simulink model "DGM_test_sim"  (R2020a)
settings: Solver=VariableStepAuto  StartTime=0.0  StopTime=smax  MaxStep=0.01  RelTol=1e-3
values from neighbouring files (symbols this model uses):
  a1 = 2    [OvereniDGMIGM.m]    (also in setup.m)
  a2 = 1.5    [OvereniDGMIGM.m]    (also in setup.m)
  a3 = 0.5    [OvereniDGMIGM.m]    (also in setup.m)
  T_1_0 = [cos(theta10), -sin(theta10), 0, a1*cos(theta10) ... (first row only)    [OvereniDGMIGM.m]    (also in setup.m)
  T_2_1 = [cos(theta20), -sin(theta20), 0, a2*cos(theta20) ... (first row only)    [OvereniDGMIGM.m]    (also in setup.m)
  T_3_2 = [cos(theta30), -sin(theta30), 0, a3*cos(theta30) ... (first row only)    [OvereniDGMIGM.m]    (also in setup.m)
undefined symbols (not defined in the file or in its folder): fi_s, fi_sample, r, R, smax, X, Y, Z
libraries: sm_lib x114, nesl_utility x58, simulink x4
(part 1 of 4)
settings Model: Creator=vilda  LastModifiedBy=Ja
settings DebuggingCC: SFMachineParentedDataDiag=error

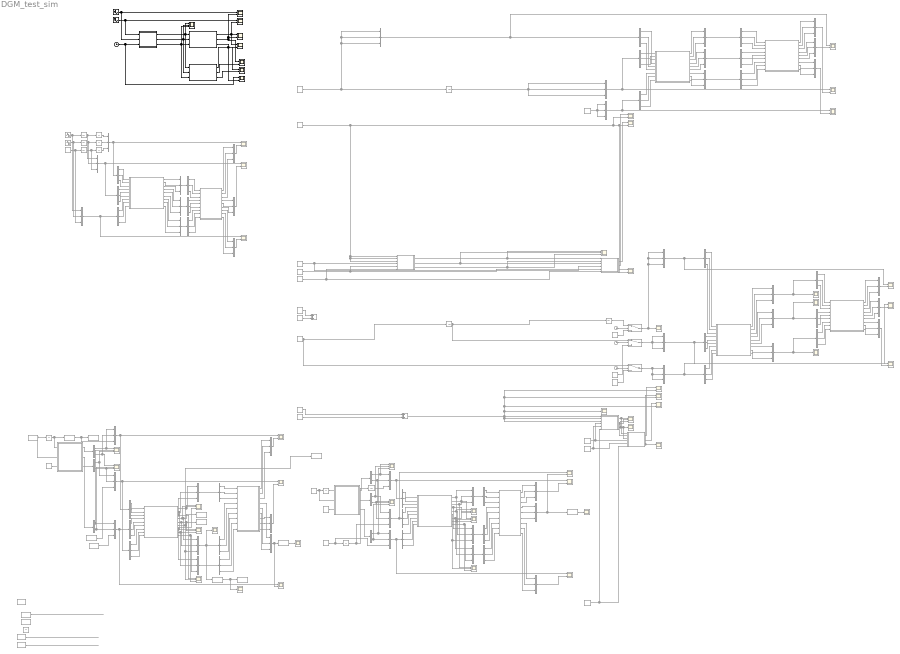
== system DGM_test_sim ==
  note: Kruhova trajektorie
  note: Rychost musi byt mensi nez vmax = 1
  note: IOKU dava manipulatoru polohu, rychlost a zrychleni v kloubech pro docileni polohy, rychlosti a zrychleni v cartezovi
  note: kloubove souradnice
  note: Generator trajektorie
  note: Generator trajektorie
  note: Rychost musi byt mensi nez vmax = 1
  note: Rychost musi byt mensi nez vmax = 1
  Add : Sum  Commented=on
  Add1 : Sum  Commented=on
  Clock : Clock  Commented=on
  Clock1 : Clock  Commented=on
  Clock2 : Clock  Commented=on
  Clock6 : Clock
  Constant{,14,16..17,21..22,24,27..28,30..31} (11 alike) : Constant  Commented=on  Value=0
  Constant10 : Constant  Commented=on  Value=0.6
  Constant11 : Constant  Commented=on  Value=fi_sample
  Constant12 : Constant  Commented=on  Value=0.1  SampleTime=-1
  Constant13 : Constant  Commented=on  Value=0.01  SampleTime=-1
  Constant15 : Constant  Commented=on
  Constant2 : Constant  Commented=on  Value=0  SampleTime=-1
  Constant23 : Constant  Commented=on
  Constant25 : Constant  Commented=on  Value=-fi_s/smax
  Constant29 : Constant  Commented=on  Value=fi_sample
  Constant3 : Constant  Commented=on  Value=a1
  Constant4 : Constant  Commented=on  Value=a2
  Constant5 : Constant  Commented=on  Value=a3
  Constant6 : Constant  Commented=on  Value=a1
  Constant7 : Constant  Commented=on  Value=a2
  Constant8 : Constant  Commented=on  Value=a3
  Demux{,1..23,27..32} (30 alike) : Demux  Commented=on  Outputs=3
  Demux{24..26,33..35} (6 alike) : Demux  Commented=on  Outputs=2
  Fcn : Fcn  Commented=on  Expr=sqrt(u(1)^2+u(2)^2+u(3)^2)
  Fcn1 : Fcn  Commented=on  Expr=sqrt(u(1)^2+u(2)^2+u(3)^2)
  Fcn2 : Fcn  Commented=on  Expr=sqrt(u(1)^2+u(2)^2+u(3)^2)
  Fcn3 : Fcn  Commented=on  Expr=fi_s - fi_s/smax*u(1)
  Integrator{,1..2,5..11,14..15,17} (13 alike) : Integrator  Commented=on
  Integrator13 : Integrator  Commented=on  InitialCondition=-pi/2/5
  MATLAB Function : MATLAB Function  Commented=on  TreatAsAtomicUnit=on
  MATLAB Function1 : MATLAB Function  Commented=on  TreatAsAtomicUnit=on
  MATLAB Function10 : MATLAB Function  Commented=on  TreatAsAtomicUnit=on
  MATLAB Function11 : MATLAB Function  Commented=on  TreatAsAtomicUnit=on
  MATLAB Function12 : MATLAB Function  Commented=on  TreatAsAtomicUnit=on
  MATLAB Function14 : MATLAB Function  Commented=on  TreatAsAtomicUnit=on
  MATLAB Function15 : MATLAB Function  Commented=on  TreatAsAtomicUnit=on
  MATLAB Function2 : MATLAB Function  Commented=on  TreatAsAtomicUnit=on
  MATLAB Function3 : MATLAB Function  Commented=on  TreatAsAtomicUnit=on
  MATLAB Function4 : MATLAB Function  Commented=on  TreatAsAtomicUnit=on
  MATLAB Function5 : MATLAB Function  TreatAsAtomicUnit=on
  MATLAB Function6 : MATLAB Function  TreatAsAtomicUnit=on
  MATLAB Function7 : MATLAB Function  Commented=on  TreatAsAtomicUnit=on
  MATLAB Function8 : MATLAB Function  Commented=on  TreatAsAtomicUnit=on
  MATLAB Function9 : MATLAB Function  Commented=on  TreatAsAtomicUnit=on
  Manipulator : Subsystem
  Manipulator1 : Subsystem  Commented=on
  Manipulator2 : Subsystem  Commented=on
  Manipulator3 : Subsystem  Commented=on
  Mux{,1..44} (45 alike) : Mux  Commented=on  Inputs=3
  Ramp3 : simulink/Sources/Ramp  Commented=on  slope=0.1  start=0  InitialOutput=0
  Ramp4 : simulink/Sources/Ramp  Commented=on  slope=-0.1  start=pi/2  InitialOutput=0
  Ramp5 : simulink/Sources/Ramp  Commented=on  slope=0.1  start=0  InitialOutput=0
  Ramp6 : simulink/Sources/Ramp  Commented=on  slope=-0.1  start=pi/2  InitialOutput=0
  Scope{,1..3,16..17,41} (7 alike) : Scope  NumInputPorts=2
  Scope{4..10,15,18..22,28..33,42..44} (22 alike) : Scope  Commented=on  NumInputPorts=2
  Scope{11,14,35..39,45..49} (12 alike) : Scope  Commented=on  NumInputPorts=3
  Scope{12..13,23..26,40,50..52} (10 alike) : Scope  Commented=on
  Scope34 : Scope  NumInputPorts=3
  Sine Wave : Sin  Commented=on  Amplitude=0.1  SampleTime=0
  Sine Wave1 : Sin  Commented=on  Amplitude=0.1  Phase=pi/2  SampleTime=0
  Sine Wave2 : Sin  SampleTime=0
  Sine Wave3 : Sin  Phase=pi/2  SampleTime=0
  Switch : Switch  Commented=on  Criteria=u2 > Threshold  Threshold=0.01
  Switch1 : Switch  Commented=on  Criteria=u2 > Threshold  Threshold=0.01
  Switch2 : Switch  Commented=on  Criteria=u2 > Threshold  Threshold=0.01
  To Workspace : ToWorkspace  Commented=on  VariableName=normdQ  SaveFormat=Structure With Time  SampleTime=-1
  To Workspace1 : ToWorkspace  Commented=on  VariableName=dQ1  SaveFormat=Structure With Time  SampleTime=-1
  To Workspace2 : ToWorkspace  Commented=on  VariableName=dQ2  SaveFormat=Structure With Time  SampleTime=-1
  To Workspace3 : ToWorkspace  Commented=on  VariableName=dQ3  SaveFormat=Structure With Time  SampleTime=-1
  To Workspace4 : ToWorkspace  Commented=on  VariableName=phi_sample  SaveFormat=Structure With Time  SampleTime=-1
  wires:
  ? -> ?
  Constant11/1 -> ?
  Constant27/1 -> ?
  Constant28/1 -> ?
  Constant17/1 -> Switch2/3
  Mux/1 -> Scope20/1, Demux3/1
  Demux6/2 -> MATLAB Function9/2(theta2)
  Constant14/1 -> Switch1/3
  Demux11/2 -> MATLAB Function10/8(ddy)
  Constant/1 -> Switch/3
  MATLAB Function10/6(theta3_dot) -> Mux16/3
  Clock2/1 -> Switch2/2
  Clock1/1 -> Switch1/2
  Demux4/2 -> MATLAB Function7/5(theta2_dot)
  Demux34/1 -> Scope47/2, Mux43/1
  MATLAB Function10/5(theta2_dot) -> Mux16/2
  MATLAB Function10/2(theta2) -> Mux15/2
  MATLAB Function9/8(ddy) -> Mux14/2
  Clock/1 -> Switch/2
  Integrator1/1 -> Switch/1
  MATLAB Function9/5(dy) -> Mux13/2
  Manipulator3/8(ddy) -> Mux41/2
  Demux8/2 -> MATLAB Function9/8(theta2_dot_dot)
  Demux8/3 -> MATLAB Function9/9(theta3_dot_dot)
  MATLAB Function9/1(x) -> Mux12/1
  MATLAB Function9/6(dphi) -> Mux13/3
  MATLAB Function10/8(theta2_dot_dot) -> Mux17/2
  MATLAB Function9/2(y) -> Mux12/2
  Mux14/1 -> Scope21/2
  Demux6/3 -> MATLAB Function9/3(theta3)
  MATLAB Function10/1(theta1) -> Mux15/1
  Demux7/2 -> MATLAB Function9/5(theta2_dot)
  Demux7/3 -> MATLAB Function9/6(theta3_dot)
  Demux10/3 -> MATLAB Function10/6(dphi)
  Demux7/1 -> MATLAB Function9/4(theta1_dot)
  MATLAB Function9/7(ddx) -> Mux14/1
  MATLAB Function10/4(theta1_dot) -> Mux16/1
  MATLAB Function14/1(theta1) -> Scope45/1, Mux36/1
  Demux11/1 -> MATLAB Function10/7(ddx)
  Demux11/3 -> MATLAB Function10/9(ddphi)
  Demux6/1 -> MATLAB Function9/1(theta1)
  Demux5/2 -> MATLAB Function7/8(theta2_dot_dot)
  MATLAB Function10/3(theta3) -> Mux15/3
  Switch2/1 -> Mux11/3, Mux11/2, Mux11/1
  Demux9/3 -> MATLAB Function10/3(phi)
  MATLAB Function12/1(theta1) -> Scope35/1, Mux18/1
  Demux10/1 -> MATLAB Function10/4(dx)
  Demux9/1 -> MATLAB Function10/1(x)
  Demux10/2 -> MATLAB Function10/5(dy)
  Demux9/2 -> MATLAB Function10/2(y)
  MATLAB Function10/9(theta3_dot_dot) -> Mux17/3
  Demux8/1 -> MATLAB Function9/7(theta1_dot_dot)
  MATLAB Function11/5(theta2_dot) -> Mux21/2
  MATLAB Function9/4(dx) -> Mux13/1
  Demux5/3 -> MATLAB Function7/9(theta3_dot_dot)
  Mux13/1 -> Scope15/2
  Demux5/1 -> MATLAB Function7/7(theta1_dot_dot)
  Demux24/2 -> Scope39/1, Mux33/2
  MATLAB Function9/9(ddphi) -> Mux14/3
  Mux12/1 -> Scope22/2
  MATLAB Function9/3(phi) -> Mux12/3
  MATLAB Function10/7(theta1_dot_dot) -> Mux17/1
  Demux4/3 -> MATLAB Function7/6(theta3_dot)
  Demux34/2 -> Scope49/2, Mux43/2
  Demux3/2 -> MATLAB Function7/2(theta2)
  Demux4/1 -> MATLAB Function7/4(theta1_dot)
  Demux/1 -> MATLAB Function8/1(x)
  Demux3/3 -> MATLAB Function7/3(theta3)
  Demux33/2 -> Scope49/1, Mux42/2
  Demux3/1 -> MATLAB Function7/1(theta1)
  Manipulator3/6(dphi) -> Mux39/3
  Mux7/1 -> Demux1/1
  Integrator9/1 -> Mux27/2
  Mux8/1 -> Demux2/1
  Demux19/2 -> MATLAB Function12/8(ddy)
  Demux2/1 -> MATLAB Function8/7(ddx)
  Manipulator2/8(ddy) -> Mux32/2
  Demux2/2 -> MATLAB Function8/8(ddy)
  Demux2/3 -> MATLAB Function8/9(ddphi)
  Demux1/1 -> MATLAB Function8/4(dx)
  Mux6/1 -> Demux/1
  Demux1/2 -> MATLAB Function8/5(dy)
  Demux25/2 -> Scope39/2, Mux34/2
  Demux1/3 -> MATLAB Function8/6(dphi)
  Demux/2 -> MATLAB Function8/2(y)
  Manipulator3/1(x) -> Mux40/1
  Manipulator2/3(phi) -> Mux31/3
  Demux/3 -> MATLAB Function8/3(phi)
  MATLAB Function7/4(dx) -> Mux7/1
  MATLAB Function7/5(dy) -> Mux7/2
  MATLAB Function7/6(dphi) -> Mux7/3
  MATLAB Function7/9(ddphi) -> Mux8/3
  MATLAB Function7/8(ddy) -> Mux8/2
  MATLAB Function7/7(ddx) -> Mux8/1
  MATLAB Function7/1(x) -> Mux6/1
  Constant23/1 -> MATLAB Function/2(v), Integrator17/1
  MATLAB Function7/2(y) -> Mux6/2
  Manipulator1/2(y) -> Mux25/2
  MATLAB Function7/3(phi) -> Mux6/3
  Mux4/1 -> Scope18/2
  MATLAB Function12/5(theta2_dot) -> Scope36/2, Mux19/2
  Mux3/1 -> Scope20/2
  Manipulator2/7(ddx) -> Mux32/1
  MATLAB Function8/9(theta3_dot_dot) -> Mux5/3
  MATLAB Function8/8(theta2_dot_dot) -> Mux5/2
  Demux35/2 -> Scope49/3, Mux44/2
  MATLAB Function8/7(theta1_dot_dot) -> Mux5/1
  MATLAB Function8/6(theta3_dot) -> Mux4/3
  MATLAB Function8/5(theta2_dot) -> Mux4/2
  Mux20/1 -> Demux17/1
  MATLAB Function8/4(theta1_dot) -> Mux4/1
  MATLAB Function/2(dXstar) -> Demux25/1
  MATLAB Function8/3(theta3) -> Mux3/3
  MATLAB Function8/2(theta2) -> Mux3/2
  Demux22/2 -> Manipulator2/8(ddQ2)
  MATLAB Function8/1(theta1) -> Mux3/1
  Mux5/1 -> Scope19/2
  Ramp5/1 -> Add1/1
  Ramp6/1 -> Add1/2
  Ramp4/1 -> Add/2
  Ramp3/1 -> Add/1
  MATLAB Function3/1(x) -> Scope8/1
  MATLAB Function3/2(y) -> Scope9/1
  MATLAB Function1/3(theta3) -> Scope6/1
  MATLAB Function1/2(theta2) -> Scope5/1
  MATLAB Function1/1(theta1) -> Scope4/1
  Switch1/1 -> Mux10/3, Mux10/1, Mux10/2
  Constant13/1 -> Switch2/1, Integrator2/1
  Integrator2/1 -> Switch1/1, Integrator1/1
  Mux10/1 -> Scope15/1, Demux10/1
  Mux16/1 -> Scope25/1, Demux7/1
  Mux9/1 -> Scope22/1, Demux9/1
  Mux17/1 -> Scope26/1, Demux8/1
  Mux11/1 -> Scope21/1, Demux11/1
  Switch/1 -> Mux9/1, Mux9/2, Mux9/3, Scope23/1
  Mux15/1 -> Scope24/1, Demux6/1
  Mux1/1 -> Scope18/1, Demux4/1
  Demux28/1 -> MATLAB Function14/7(ddx)
  Constant2/1 -> Mux2/3, Mux2/1, Mux2/2
  Mux2/1 -> Scope19/1, Demux5/1
  Manipulator3/5(dy) -> Mux39/2
  Integrator/1 -> Mux/3, Mux/1, Mux/2
  Constant12/1 -> Mux1/1, Mux1/2, Mux1/3, Integrator/1
  MATLAB Function2/1(x) -> Scope14/1, MATLAB Function1/1(x)
  MATLAB Function3/3(phi) -> Scope10/1, Scope7/1
  MATLAB Function4/1(theta1) -> Scope11/1, MATLAB Function3/1(theta1)
  MATLAB Function4/2(theta2) -> Scope11/2, MATLAB Function3/2(theta2)
  Manipulator1/3(phi) -> Mux25/3
  Constant8/1 -> MATLAB Function3/6(a3), MATLAB Function4/6(a3)
  Constant7/1 -> MATLAB Function3/5(a2), MATLAB Function4/5(a2)
  Constant16/1 -> MATLAB Function15/3(a)
  Constant6/1 -> MATLAB Function3/4(a1), MATLAB Function4/4(a1)
  MATLAB Function4/3(theta3) -> Scope12/1, MATLAB Function3/3(theta3), Scope11/3
  Add/1 -> MATLAB Function4/3(phi), MATLAB Function4/2(y), Scope10/2, Scope8/2, Scope9/2, Scope13/1, MATLAB Function4/1(x)
  MATLAB Function2/3(phi) -> Scope14/3, MATLAB Function1/3(phi)
  MATLAB Function2/2(y) -> Scope14/2, MATLAB Function1/2(y)
  Manipulator2/9(ddphi) -> Mux32/3
  Constant4/1 -> MATLAB Function2/5(a2), MATLAB Function1/5(a2)
  Constant3/1 -> MATLAB Function2/4(a1), MATLAB Function1/4(a1)
  Integrator10/1 -> Mux27/3
  Constant10/1 -> MATLAB Function2/3(theta3), MATLAB Function2/2(theta2), MATLAB Function2/1(theta1), Scope4/2, Scope6/2, Scope5/2
  Constant5/1 -> MATLAB Function2/6(a3), MATLAB Function1/6(a3)
  Fcn/1 -> Scope40/1
  Constant24/1 -> MATLAB Function/3(a)
  MATLAB Function6/2(Q2) -> Scope34/2, Manipulator/2(Q2), MATLAB Function5/2(Q2)
  Integrator17/1 -> MATLAB Function/1(s)
  MATLAB Function/1(Xstar) -> Demux24/1
  MATLAB Function/3(ddXstar) -> Demux26/1
  Manipulator2/1(x) -> Mux31/1
  Demux21/1 -> Manipulator2/4(dQ1)
  Demux23/1 -> Manipulator2/1(Q1)
  Demux19/3 -> MATLAB Function12/9(ddphi)
  Mux18/1 -> Demux23/1
  Demux18/2 -> MATLAB Function12/5(dy)
  Demux20/2 -> MATLAB Function12/2(y)
  Demux23/2 -> Manipulator2/2(Q2)
  Manipulator2/4(dx) -> Mux30/1
  Demux12/2 -> MATLAB Function11/5(dy)
  Demux18/3 -> MATLAB Function12/6(dphi)
  Mux23/1 -> Demux22/1
  Demux18/1 -> MATLAB Function12/4(dx)
  Demux19/1 -> MATLAB Function12/7(ddx)
  Demux20/1 -> MATLAB Function12/1(x)
  Demux20/3 -> MATLAB Function12/3(phi)
  Manipulator2/2(y) -> Mux31/2
  Manipulator2/6(dphi) -> Mux30/3
  Mux36/1 -> Demux32/1
  Demux22/3 -> Manipulator2/9(ddQ3)
  Mux19/1 -> Demux21/1
  Mux31/1 -> Scope31/2
  Mux32/1 -> Scope33/2
  Demux21/3 -> Manipulator2/6(dQ3)
  Demux23/3 -> Manipulator2/3(Q3)
  Demux22/1 -> Manipulator2/7(ddQ1)
  MATLAB Function15/3(ddXstar) -> Demux35/1
  Demux21/2 -> Manipulator2/5(dQ2)
  Integrator11/1 -> Mux33/3
  Manipulator3/2(y) -> Mux40/2
  Manipulator2/5(dy) -> Mux30/2
  Constant22/1 -> Integrator14/1, Mux35/3
  Demux26/2 -> Scope39/3, Mux35/2
  MATLAB Function6/3(Q3) -> Scope34/3, Manipulator/3(Q3), MATLAB Function5/3(Q3)
  Demux26/1 -> Scope37/3, Mux35/1
  Demux24/1 -> Scope37/1, Mux33/1
  Demux25/1 -> Scope37/2, Mux34/1
  MATLAB Function12/7(theta1_dot_dot) -> Scope35/3, Mux23/1
  MATLAB Function14/8(theta2_dot_dot) -> Scope46/3, Mux38/2
  MATLAB Function12/3(theta3) -> Scope38/1, Mux18/3
  MATLAB Function12/4(theta1_dot) -> Scope35/2, Mux19/1
  MATLAB Function12/6(theta3_dot) -> Scope38/2, Mux19/3
  MATLAB Function12/2(theta2) -> Scope36/1, Mux18/2
  MATLAB Function12/8(theta2_dot_dot) -> Scope36/3, Mux23/2
  MATLAB Function12/9(theta3_dot_dot) -> Scope38/3, Mux23/3
  Integrator14/1 -> Integrator11/1, Mux34/3
  Mux30/1 -> Scope32/2, Fcn/1
  Mux27/1 -> Scope28/1, Demux14/1
  Mux35/1 -> Scope33/1, Demux19/1
  Mux34/1 -> Scope32/1, Demux18/1
  Mux33/1 -> Scope31/1, Demux20/1
  Manipulator/3(phi) -> Scope17/2, Scope3/1
  Constant30/1 -> Mux44/3
  Constant25/1 -> Mux43/3
  MATLAB Function15/2(dXstar) -> Demux34/1
  MATLAB Function15/1(Xstar) -> Demux33/1
  Demux29/1 -> MATLAB Function14/1(x)
  Manipulator3/9(ddphi) -> Mux41/3
  Demux32/3 -> Manipulator3/3(Q3)
  Demux32/1 -> Manipulator3/1(Q1)
  Demux31/3 -> Manipulator3/9(ddQ3)
  Mux40/1 -> Scope42/2
  Demux31/2 -> Manipulator3/8(ddQ2)
  Demux29/3 -> MATLAB Function14/3(phi)
  Demux27/1 -> MATLAB Function14/4(dx)
  Demux31/1 -> Manipulator3/7(ddQ1)
  Manipulator3/3(phi) -> Mux40/3
  MATLAB Function11/3(theta3) -> Mux20/3
  Demux27/3 -> MATLAB Function14/6(dphi)
  Manipulator3/7(ddx) -> Mux41/1
  Demux32/2 -> Manipulator3/2(Q2)
  Demux29/2 -> MATLAB Function14/2(y)
  Demux27/2 -> MATLAB Function14/5(dy)
  Mux41/1 -> Scope44/2
  Demux30/1 -> Manipulator3/4(dQ1)
  Demux28/2 -> MATLAB Function14/8(ddy)
  Manipulator3/4(dx) -> Mux39/1
  Demux30/3 -> Manipulator3/6(dQ3)
  Mux38/1 -> Demux31/1
  Fcn1/1 -> Scope50/1
  Manipulator1/6(dphi) -> Mux24/3
  Demux28/3 -> MATLAB Function14/9(ddphi)
  Demux30/2 -> Manipulator3/5(dQ2)
  Fcn3/1 -> To Workspace4/1, Mux42/3
  Mux24/1 -> Scope29/2
  Integrator15/1 -> Fcn3/1, MATLAB Function15/1(s)
  Mux37/1 -> Fcn2/1, Scope52/1, Demux30/1
  Fcn2/1 -> To Workspace/1, Scope51/1
  MATLAB Function14/5(theta2_dot) -> To Workspace2/1, Scope46/2, Mux37/2
  Mux44/1 -> Scope44/1, Demux28/1
  MATLAB Function14/9(theta3_dot_dot) -> Scope48/3, Mux38/3
  Mux43/1 -> Scope43/1, Demux27/1
  Mux39/1 -> Scope43/2, Fcn1/1
  Mux42/1 -> Scope42/1, Demux29/1
  Demux33/1 -> Scope47/1, Mux42/1
  MATLAB Function14/6(theta3_dot) -> Scope48/2, Mux37/3, To Workspace3/1
  MATLAB Function14/3(theta3) -> Scope48/1, Mux36/3
  Constant15/1 -> Integrator15/1, MATLAB Function15/2(v)
  Demux17/1 -> Manipulator1/1(Q1)
  MATLAB Function14/2(theta2) -> Scope46/1, Mux36/2
  MATLAB Function14/7(theta1_dot_dot) -> Scope45/3, Mux38/1
  MATLAB Function11/4(theta1_dot) -> Mux21/1
  Demux35/1 -> Scope47/3, Mux44/1
  MATLAB Function14/4(theta1_dot) -> To Workspace1/1, Mux37/1, Scope45/2
  Integrator8/1 -> Mux27/1
  Manipulator1/9(ddphi) -> Mux26/3
  Manipulator1/7(ddx) -> Mux26/1
  Manipulator1/8(ddy) -> Mux26/2
  Mux26/1 -> Scope30/2
  Manipulator1/4(dx) -> Mux24/1
  Manipulator1/5(dy) -> Mux24/2
  Mux25/1 -> Scope28/2
  Manipulator1/1(x) -> Mux25/1
  Mux22/1 -> Demux16/1
  Demux16/2 -> Manipulator1/8(ddQ2)
  Mux21/1 -> Demux15/1
  Demux17/2 -> Manipulator1/2(Q2)
  Demux17/3 -> Manipulator1/3(Q3)
  Demux16/3 -> Manipulator1/9(ddQ3)
  Demux15/2 -> Manipulator1/5(dQ2)
  Demux15/1 -> Manipulator1/4(dQ1)
  Demux15/3 -> Manipulator1/6(dQ3)
  Demux16/1 -> Manipulator1/7(ddQ1)
  MATLAB Function11/9(theta3_dot_dot) -> Mux22/3
  MATLAB Function11/8(theta2_dot_dot) -> Mux22/2
  Demux14/2 -> MATLAB Function11/2(y)
  Demux14/1 -> MATLAB Function11/1(x)
  Demux14/3 -> MATLAB Function11/3(phi)
  Demux12/1 -> MATLAB Function11/4(dx)
  Demux12/3 -> MATLAB Function11/6(dphi)
  Demux13/2 -> MATLAB Function11/8(ddy)
  Demux13/1 -> MATLAB Function11/7(ddx)
  MATLAB Function11/1(theta1) -> Mux20/1
  MATLAB Function11/7(theta1_dot_dot) -> Mux22/1
  MATLAB Function11/2(theta2) -> Mux20/2
  MATLAB Function5/2(y) -> Scope2/2
  Demux13/3 -> MATLAB Function11/9(ddphi)
  MATLAB Function11/6(theta3_dot) -> Mux21/3
  Integrator6/1 -> Mux28/2, Integrator9/1
  Integrator5/1 -> Integrator8/1, Mux28/1
  Constant21/1 -> Integrator7/1, Mux29/3
  Integrator7/1 -> Integrator10/1, Mux28/3
  Sine Wave/1 -> Integrator5/1, Mux29/1
  Sine Wave1/1 -> Integrator6/1, Mux29/2
  Mux29/1 -> Scope30/1, Demux13/1
  Mux28/1 -> Scope29/1, Demux12/1
  MATLAB Function5/1(x) -> Scope1/2
  MATLAB Function5/3(phi) -> Scope3/2
  MATLAB Function6/1(Q1) -> Scope34/1, Manipulator/1(Q1), MATLAB Function5/1(Q1)
  Clock6/1 -> Scope17/1, MATLAB Function6/3(phi)
  Sine Wave3/1 -> Scope16/1, MATLAB Function6/2(y)
  Sine Wave2/1 -> Scope/1, MATLAB Function6/1(x)
  Manipulator/2(y) -> Scope16/2, Scope41/2, Scope2/1
  Manipulator/1(x) -> Scope1/1, Scope41/1, Scope/2

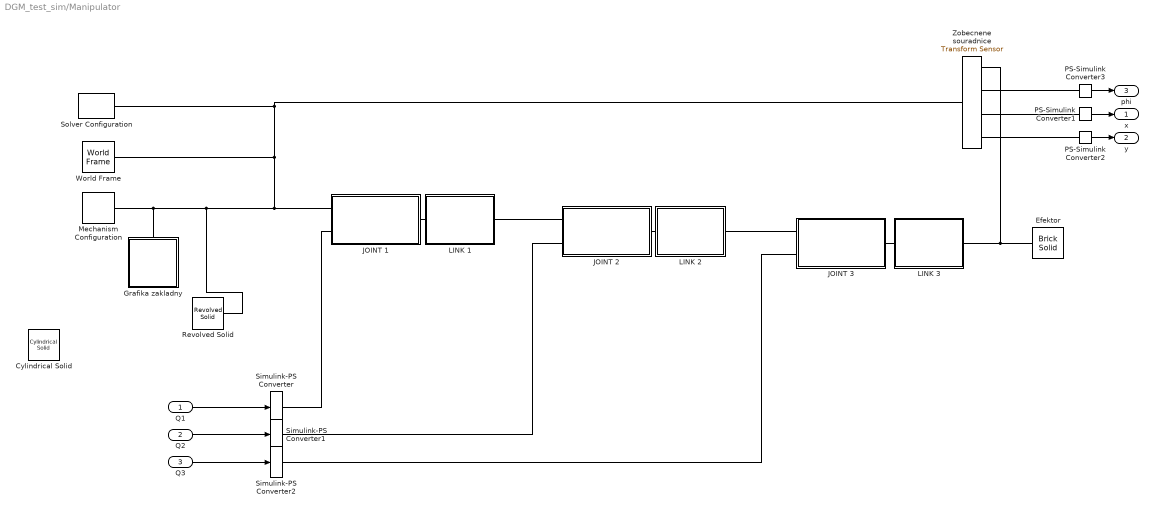
== system DGM_test_sim/Manipulator ==
  Q1 : Inport
  Q2 : Inport  Port=2
  Q3 : Inport  Port=3
  Cylindrical Solid : sm_lib/Body Elements/Cylindrical Solid  GraphicAmbientColor=[0.15 0.15 0.15 1.0]  BasedOnType=Density  CenterOfMass=[0 0 0]  CenterOfMassUnits=m  GraphicDiffuseColor=[0.5 0.5 0.5]  CylinderLength=1  CylinderLengthUnits=m  CylinderRadius=1  CylinderRadiusUnits=m  Density=1000  DensityUnits=kg/m^3  DoExposeReferenceFrame=on  GraphicEmissiveColor=[0.0 0.0 0.0 1.0]  ExportEntireGeometry=off  SerializedFrames=<Frames/>  MarkerShape=Sphere  MarkerSize=10  GraphicType=FromGeometry  InertiaType=CalculateFromGeometry  Mass=1  MassUnits=kg  MomentsOfInertia=[1 1 1]  MomentsOfInertiaUnits=kg*m^2  GraphicOpacity=1.0  ProductsOfInertia=[0 0 0]  ProductsOfInertiaUnits=kg*m^2  GraphicShininess=75  GraphicSpecularColor=[0.5 0.5 0.5 1.0]  GraphicVisPropType=SimpleVisualProperties
  Efektor : sm_lib/Body Elements/Brick Solid  GraphicAmbientColor=[0.15 0.15 0.15 1.0]  BasedOnType=Density  BrickDimensions=[0.1 0.1 0.1]  BrickDimensionUnits=m  CenterOfMass=[0 0 0]  CenterOfMassUnits=m  GraphicDiffuseColor=[0.5 0.5 0.5]  Density=1000  DensityUnits=kg/m^3  DoExposeReferenceFrame=on  GraphicEmissiveColor=[0.0 0.0 0.0 1.0]  ExportEntireGeometry=off  SerializedFrames=<Frames/>  MarkerShape=Sphere  MarkerSize=10  GraphicType=FromGeometry  InertiaType=CalculateFromGeometry  Mass=1  MassUnits=kg  MomentsOfInertia=[1 1 1]  MomentsOfInertiaUnits=kg*m^2  GraphicOpacity=1.0  ProductsOfInertia=[0 0 0]  ProductsOfInertiaUnits=kg*m^2  GraphicShininess=75  GraphicSpecularColor=[0.5 0.5 0.5 1.0]  GraphicVisPropType=SimpleVisualProperties
  Grafika zakladny : Subsystem
  JOINT 1 : Subsystem
  JOINT 2 : Subsystem
  JOINT 3 : Subsystem
  LINK 1 : Subsystem
  LINK 2 : Subsystem
  LINK 3 : Subsystem
  Mechanism Configuration : sm_lib/Utilities/Mechanism Configuration  UniformGravity=Constant  GravityVector=[0 0 -9.80665]  GravityUnits=m/s^2  LinearizationDelta=0.001
  PS-Simulink Converter1 : nesl_utility/PS-Simulink Converter  PhysicalDomain=network_engine_domain  SubClassName=ps_output  LeftPortType=input  RightPortType=output  PseudoPeriodic=off  Frequencies=[]  Unit=inherit  AffineConversion=off
      settings: SourceProductBaseCode=PW,SS
  PS-Simulink Converter2 : nesl_utility/PS-Simulink Converter  PhysicalDomain=network_engine_domain  SubClassName=ps_output  LeftPortType=input  RightPortType=output  PseudoPeriodic=off  Frequencies=[]  Unit=inherit  AffineConversion=off
      settings: SourceProductBaseCode=PW,SS
  PS-Simulink Converter3 : nesl_utility/PS-Simulink Converter  PhysicalDomain=network_engine_domain  SubClassName=ps_output  LeftPortType=input  RightPortType=output  PseudoPeriodic=off  Frequencies=[]  Unit=inherit  AffineConversion=off
      settings: SourceProductBaseCode=PW,SS
  Revolved Solid : sm_lib/Body Elements/Revolved Solid  GraphicAmbientColor=[0.15 0.15 0.15 1.0]  BasedOnType=Density  CenterOfMass=[0 0 0]  CenterOfMassUnits=m  GraphicDiffuseColor=[0.5 0.5 0.5]  ExportConvexHullGeometry=off  Density=1000  DensityUnits=kg/m^3  DoExposeReferenceFrame=on  GraphicEmissiveColor=[0.0 0.0 0.0 1.0]  ExportEntireGeometry=off  SerializedFrames=<Frames/>  MarkerShape=Sphere  MarkerSize=10  GraphicType=FromGeometry  InertiaType=CalculateFromGeometry  Mass=1  MassUnits=kg  MomentsOfInertia=[1 1 1]  MomentsOfInertiaUnits=kg*m^2  GraphicOpacity=0.2  ProductsOfInertia=[0 0 0]  ProductsOfInertiaUnits=kg*m^2  RevolutionCrossSection=[r 0.01; r -0.01; R -0.01; R 0.01]  RevolutionCrossSectionUnits=m  RevolutionAngle=180  RevolutionAngleUnits=deg  RevolutionExtent=Full  GraphicShininess=75  GraphicSpecularColor=[0.5 0.5 0.5 1.0]  GraphicVisPropType=SimpleVisualProperties
  Simulink-PS Converter : nesl_utility/Simulink-PS Converter  PhysicalDomain=network_engine_domain  SubClassName=ps_input  LeftPortType=input  RightPortType=output  PseudoPeriodic=off  Frequencies=[]  NoiseDistribution=none  NoiseParameters=[]  Unit=1  AffineConversion=off  FilteringAndDerivatives=filter  SimscapeFilterOrder=2  InputFilterTimeConstant=0.001  UdotUserProvided=0
      settings: SourceProductBaseCode=PW,SS
  Simulink-PS Converter1 : nesl_utility/Simulink-PS Converter  PhysicalDomain=network_engine_domain  SubClassName=ps_input  LeftPortType=input  RightPortType=output  PseudoPeriodic=off  Frequencies=[]  NoiseDistribution=none  NoiseParameters=[]  Unit=1  AffineConversion=off  FilteringAndDerivatives=filter  SimscapeFilterOrder=2  InputFilterTimeConstant=0.001  UdotUserProvided=0
      settings: SourceProductBaseCode=PW,SS
  Simulink-PS Converter2 : nesl_utility/Simulink-PS Converter  PhysicalDomain=network_engine_domain  SubClassName=ps_input  LeftPortType=input  RightPortType=output  PseudoPeriodic=off  Frequencies=[]  NoiseDistribution=none  NoiseParameters=[]  Unit=1  AffineConversion=off  FilteringAndDerivatives=filter  SimscapeFilterOrder=2  InputFilterTimeConstant=0.001  UdotUserProvided=0
      settings: SourceProductBaseCode=PW,SS
  Solver Configuration : nesl_utility/Solver Configuration  PhysicalDomain=network_engine_domain  SubClassName=solver  LeftPortType=input  RightPortType=generic  Tones=[]  Harmonics=[]  SimulateNoise=off  Profile=off  UseLocalSampling=off  EnableSwitchedLinearOptims=on  FrequencyDomain=off  UseCCode=off  RelTol=0.001  AbsTol=1e-06  MinStep=1e-09  ToWorkspace=off  RevertToSquareIcSolve=off  NumHomotopyIterations=100  PhasorMode=off  PhasorModeNumHarmonics=1  DoDC=off  ResidualTolerance=1e-09  UseLocalSolver=off  LocalSolverChoice=NE_BACKWARD_EULER_ADVANCER  LocalSolverSampleTime=0.001  DoFixedCost=off  MaxNonlinIter=3  MaxModeIter=2  LinearAlgebra=auto  EquationFormulation=NE_TIME_EF  DelaysMemoryBudget=1024  AutomaticFiltering=on  FilteringTimeConstant=0.001  PartitionStorageMethod=AS_NEEDED  PartitionMemoryBudget=1024  PartitionMethod=ROBUST
      settings: SourceProductBaseCode=PW,SS
  World Frame : sm_lib/Frames and Transforms/World Frame
  Zobecnene souradnice : sm_lib/Frames and Transforms/Transform Sensor  MeasurementFrame=World  SenseAngle=on  SenseAxis=off  SenseAngle1=off  SenseAngle2=off  SenseAngle3=off  SenseQ=off  SenseR=off  SenseOmegaX=off  SenseOmegaY=off  SenseOmegaZ=off  SenseOmega1=off  SenseOmega2=off  SenseOmega3=off  SenseQDot=off  SenseRDot=off  SenseAlphaX=off  SenseAlphaY=off  SenseAlphaZ=off  SenseAlpha1=off  SenseAlpha2=off  SenseAlpha3=off  SenseQDDot=off  SenseRDDot=off  SenseX=on  SenseY=on  SenseZ=off  SenseRad=off  SenseAzim=off  SenseDist=off  SenseInc=off  SenseXDot=off  SenseYDot=off  SenseZDot=off  SenseRadDot=off  SenseAzimDot=off  SenseDistDot=off  SenseIncDot=off  SenseXDDot=off  SenseYDDot=off  SenseZDDot=off  SenseRadDDot=off  SenseAzimDDot=off  SenseDistDDot=off  SenseIncDDot=off
  x : Outport
  y : Outport  Port=2
  phi : Outport  Port=3
  wires:
  PS-Simulink Converter1/1 -> x/1
  PS-Simulink Converter2/1 -> y/1
  PS-Simulink Converter3/1 -> phi/1
  Q1/1 -> Simulink-PS Converter/1
  Q2/1 -> Simulink-PS Converter1/1
  Q3/1 -> Simulink-PS Converter2/1
  connections:
  Zobecnene souradnice/RConn1 -- Efektor/RConn1 -- LINK 3/RConn1
  Zobecnene souradnice/RConn2 -- PS-Simulink Converter3/LConn1
  Zobecnene souradnice/RConn4 -- PS-Simulink Converter2/LConn1
  PS-Simulink Converter1/LConn1 -- Zobecnene souradnice/RConn3
  Solver Configuration/RConn1 -- Revolved Solid/RConn1 -- Mechanism Configuration/RConn1 -- Grafika zakladny/LConn1 -- JOINT 1/LConn1 -- World Frame/RConn1 -- Zobecnene souradnice/LConn1
  LINK 1/LConn1 -- JOINT 1/RConn1
  JOINT 1/LConn2 -- Simulink-PS Converter/RConn1
  JOINT 2/LConn1 -- LINK 1/RConn1
  JOINT 2/RConn1 -- LINK 2/LConn1
  Simulink-PS Converter1/RConn1 -- JOINT 2/LConn2
  JOINT 3/LConn1 -- LINK 2/RConn1
  JOINT 3/RConn1 -- LINK 3/LConn1
  Simulink-PS Converter2/RConn1 -- JOINT 3/LConn2

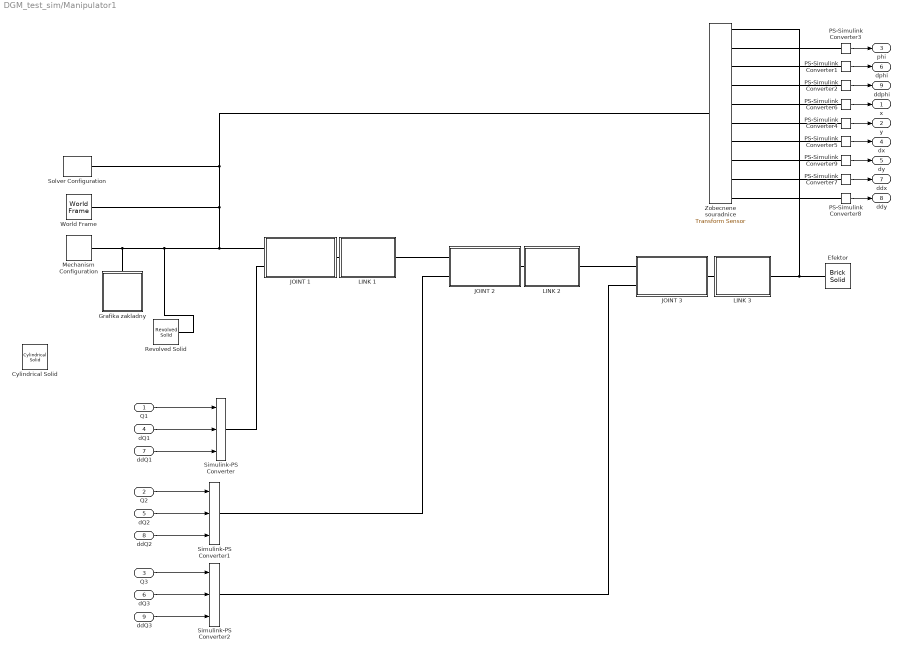
== system DGM_test_sim/Manipulator1 ==
  Q1 : Inport
  Q2 : Inport  Port=2
  Q3 : Inport  Port=3
  dQ1 : Inport  Port=4
  dQ2 : Inport  Port=5
  dQ3 : Inport  Port=6
  ddQ1 : Inport  Port=7
  ddQ2 : Inport  Port=8
  ddQ3 : Inport  Port=9
  Cylindrical Solid : sm_lib/Body Elements/Cylindrical Solid  GraphicAmbientColor=[0.15 0.15 0.15 1.0]  BasedOnType=Density  CenterOfMass=[0 0 0]  CenterOfMassUnits=m  GraphicDiffuseColor=[0.5 0.5 0.5]  CylinderLength=1  CylinderLengthUnits=m  CylinderRadius=1  CylinderRadiusUnits=m  Density=1000  DensityUnits=kg/m^3  DoExposeReferenceFrame=on  GraphicEmissiveColor=[0.0 0.0 0.0 1.0]  ExportEntireGeometry=off  SerializedFrames=<Frames/>  MarkerShape=Sphere  MarkerSize=10  GraphicType=FromGeometry  InertiaType=CalculateFromGeometry  Mass=1  MassUnits=kg  MomentsOfInertia=[1 1 1]  MomentsOfInertiaUnits=kg*m^2  GraphicOpacity=1.0  ProductsOfInertia=[0 0 0]  ProductsOfInertiaUnits=kg*m^2  GraphicShininess=75  GraphicSpecularColor=[0.5 0.5 0.5 1.0]  GraphicVisPropType=SimpleVisualProperties
  Efektor : sm_lib/Body Elements/Brick Solid  GraphicAmbientColor=[0.15 0.15 0.15 1.0]  BasedOnType=Density  BrickDimensions=[0.1 0.1 0.1]  BrickDimensionUnits=m  CenterOfMass=[0 0 0]  CenterOfMassUnits=m  GraphicDiffuseColor=[0.5 0.5 0.5]  Density=1000  DensityUnits=kg/m^3  DoExposeReferenceFrame=on  GraphicEmissiveColor=[0.0 0.0 0.0 1.0]  ExportEntireGeometry=off  SerializedFrames=<Frames/>  MarkerShape=Sphere  MarkerSize=10  GraphicType=FromGeometry  InertiaType=CalculateFromGeometry  Mass=1  MassUnits=kg  MomentsOfInertia=[1 1 1]  MomentsOfInertiaUnits=kg*m^2  GraphicOpacity=1.0  ProductsOfInertia=[0 0 0]  ProductsOfInertiaUnits=kg*m^2  GraphicShininess=75  GraphicSpecularColor=[0.5 0.5 0.5 1.0]  GraphicVisPropType=SimpleVisualProperties
  Grafika zakladny : Subsystem
  JOINT 1 : Subsystem
  JOINT 2 : Subsystem
  JOINT 3 : Subsystem
  LINK 1 : Subsystem
  LINK 2 : Subsystem
  LINK 3 : Subsystem
  Mechanism Configuration : sm_lib/Utilities/Mechanism Configuration  UniformGravity=Constant  GravityVector=[0 0 -9.80665]  GravityUnits=m/s^2  LinearizationDelta=0.001
  PS-Simulink Converter{1..9} (9 alike) : nesl_utility/PS-Simulink Converter  PhysicalDomain=network_engine_domain  SubClassName=ps_output  LeftPortType=input  RightPortType=output  PseudoPeriodic=off  Frequencies=[]  Unit=inherit  AffineConversion=off
      settings: SourceProductBaseCode=PW,SS
  Revolved Solid : sm_lib/Body Elements/Revolved Solid  GraphicAmbientColor=[0.15 0.15 0.15 1.0]  BasedOnType=Density  CenterOfMass=[0 0 0]  CenterOfMassUnits=m  GraphicDiffuseColor=[0.5 0.5 0.5]  ExportConvexHullGeometry=off  Density=1000  DensityUnits=kg/m^3  DoExposeReferenceFrame=on  GraphicEmissiveColor=[0.0 0.0 0.0 1.0]  ExportEntireGeometry=off  SerializedFrames=<Frames/>  MarkerShape=Sphere  MarkerSize=10  GraphicType=FromGeometry  InertiaType=CalculateFromGeometry  Mass=1  MassUnits=kg  MomentsOfInertia=[1 1 1]  MomentsOfInertiaUnits=kg*m^2  GraphicOpacity=0.2  ProductsOfInertia=[0 0 0]  ProductsOfInertiaUnits=kg*m^2  RevolutionCrossSection=[r 0.01; r -0.01; R -0.01; R 0.01]  RevolutionCrossSectionUnits=m  RevolutionAngle=180  RevolutionAngleUnits=deg  RevolutionExtent=Full  GraphicShininess=75  GraphicSpecularColor=[0.5 0.5 0.5 1.0]  GraphicVisPropType=SimpleVisualProperties
  Simulink-PS Converter : nesl_utility/Simulink-PS Converter  PhysicalDomain=network_engine_domain  SubClassName=ps_input  LeftPortType=input  RightPortType=output  PseudoPeriodic=off  Frequencies=[]  NoiseDistribution=none  NoiseParameters=[]  Unit=1  AffineConversion=off  FilteringAndDerivatives=provide  SimscapeFilterOrder=2  InputFilterTimeConstant=0.001  UdotUserProvided=2
      settings: SourceProductBaseCode=PW,SS
  Simulink-PS Converter1 : nesl_utility/Simulink-PS Converter  PhysicalDomain=network_engine_domain  SubClassName=ps_input  LeftPortType=input  RightPortType=output  PseudoPeriodic=off  Frequencies=[]  NoiseDistribution=none  NoiseParameters=[]  Unit=1  AffineConversion=off  FilteringAndDerivatives=provide  SimscapeFilterOrder=2  InputFilterTimeConstant=0.001  UdotUserProvided=2
      settings: SourceProductBaseCode=PW,SS
  Simulink-PS Converter2 : nesl_utility/Simulink-PS Converter  PhysicalDomain=network_engine_domain  SubClassName=ps_input  LeftPortType=input  RightPortType=output  PseudoPeriodic=off  Frequencies=[]  NoiseDistribution=none  NoiseParameters=[]  Unit=1  AffineConversion=off  FilteringAndDerivatives=provide  SimscapeFilterOrder=2  InputFilterTimeConstant=0.001  UdotUserProvided=2
      settings: SourceProductBaseCode=PW,SS
  Solver Configuration : nesl_utility/Solver Configuration  PhysicalDomain=network_engine_domain  SubClassName=solver  LeftPortType=input  RightPortType=generic  Tones=[]  Harmonics=[]  SimulateNoise=off  Profile=off  UseLocalSampling=off  EnableSwitchedLinearOptims=on  FrequencyDomain=off  UseCCode=off  RelTol=0.001  AbsTol=1e-06  MinStep=1e-09  ToWorkspace=off  RevertToSquareIcSolve=off  NumHomotopyIterations=100  PhasorMode=off  PhasorModeNumHarmonics=1  DoDC=off  ResidualTolerance=1e-09  UseLocalSolver=off  LocalSolverChoice=NE_BACKWARD_EULER_ADVANCER  LocalSolverSampleTime=0.001  DoFixedCost=off  MaxNonlinIter=3  MaxModeIter=2  LinearAlgebra=auto  EquationFormulation=NE_TIME_EF  DelaysMemoryBudget=1024  AutomaticFiltering=on  FilteringTimeConstant=0.001  PartitionStorageMethod=AS_NEEDED  PartitionMemoryBudget=1024  PartitionMethod=ROBUST
      settings: SourceProductBaseCode=PW,SS
  World Frame : sm_lib/Frames and Transforms/World Frame
  Zobecnene souradnice : sm_lib/Frames and Transforms/Transform Sensor  MeasurementFrame=World  SenseAngle=on  SenseAxis=off  SenseAngle1=off  SenseAngle2=off  SenseAngle3=off  SenseQ=off  SenseR=off  SenseOmegaX=off  SenseOmegaY=off  SenseOmegaZ=on  SenseOmega1=off  SenseOmega2=off  SenseOmega3=off  SenseQDot=off  SenseRDot=off  SenseAlphaX=off  SenseAlphaY=off  SenseAlphaZ=on  SenseAlpha1=off  SenseAlpha2=off  SenseAlpha3=off  SenseQDDot=off  SenseRDDot=off  SenseX=on  SenseY=on  SenseZ=off  SenseRad=off  SenseAzim=off  SenseDist=off  SenseInc=off  SenseXDot=on  SenseYDot=on  SenseZDot=off  SenseRadDot=off  SenseAzimDot=off  SenseDistDot=off  SenseIncDot=off  SenseXDDot=on  SenseYDDot=on  SenseZDDot=off  SenseRadDDot=off  SenseAzimDDot=off  SenseDistDDot=off  SenseIncDDot=off
  x : Outport
  y : Outport  Port=2
  phi : Outport  Port=3
  dx : Outport  Port=4
  dy : Outport  Port=5
  dphi : Outport  Port=6
  ddx : Outport  Port=7
  ddy : Outport  Port=8
  ddphi : Outport  Port=9
  wires:
  PS-Simulink Converter2/1 -> ddphi/1
  dQ1/1 -> Simulink-PS Converter/2
  Q1/1 -> Simulink-PS Converter/1
  ddQ1/1 -> Simulink-PS Converter/3
  Q2/1 -> Simulink-PS Converter1/1
  ddQ2/1 -> Simulink-PS Converter1/3
  Q3/1 -> Simulink-PS Converter2/1
  dQ3/1 -> Simulink-PS Converter2/2
  ddQ3/1 -> Simulink-PS Converter2/3
  dQ2/1 -> Simulink-PS Converter1/2
  PS-Simulink Converter6/1 -> x/1
  PS-Simulink Converter5/1 -> dx/1
  PS-Simulink Converter7/1 -> ddx/1
  PS-Simulink Converter4/1 -> y/1
  PS-Simulink Converter3/1 -> phi/1
  PS-Simulink Converter1/1 -> dphi/1
  PS-Simulink Converter9/1 -> dy/1
  PS-Simulink Converter8/1 -> ddy/1
  connections:
  Zobecnene souradnice/RConn1 -- Efektor/RConn1 -- LINK 3/RConn1
  Zobecnene souradnice/RConn2 -- PS-Simulink Converter3/LConn1
  Zobecnene souradnice/RConn4 -- PS-Simulink Converter2/LConn1
  PS-Simulink Converter1/LConn1 -- Zobecnene souradnice/RConn3
  Solver Configuration/RConn1 -- Revolved Solid/RConn1 -- Mechanism Configuration/RConn1 -- Grafika zakladny/LConn1 -- JOINT 1/LConn1 -- World Frame/RConn1 -- Zobecnene souradnice/LConn1
  LINK 1/LConn1 -- JOINT 1/RConn1
  JOINT 1/LConn2 -- Simulink-PS Converter/RConn1
  JOINT 2/LConn1 -- LINK 1/RConn1
  JOINT 2/RConn1 -- LINK 2/LConn1
  JOINT 3/LConn1 -- LINK 2/RConn1
  JOINT 3/RConn1 -- LINK 3/LConn1
  Simulink-PS Converter1/RConn1 -- JOINT 2/LConn2
  Simulink-PS Converter2/RConn1 -- JOINT 3/LConn2
  Zobecnene souradnice/RConn6 -- PS-Simulink Converter4/LConn1
  Zobecnene souradnice/RConn5 -- PS-Simulink Converter6/LConn1
  Zobecnene souradnice/RConn7 -- PS-Simulink Converter5/LConn1
  Zobecnene souradnice/RConn9 -- PS-Simulink Converter7/LConn1
  Zobecnene souradnice/RConn8 -- PS-Simulink Converter9/LConn1
  Zobecnene souradnice/RConn10 -- PS-Simulink Converter8/LConn1

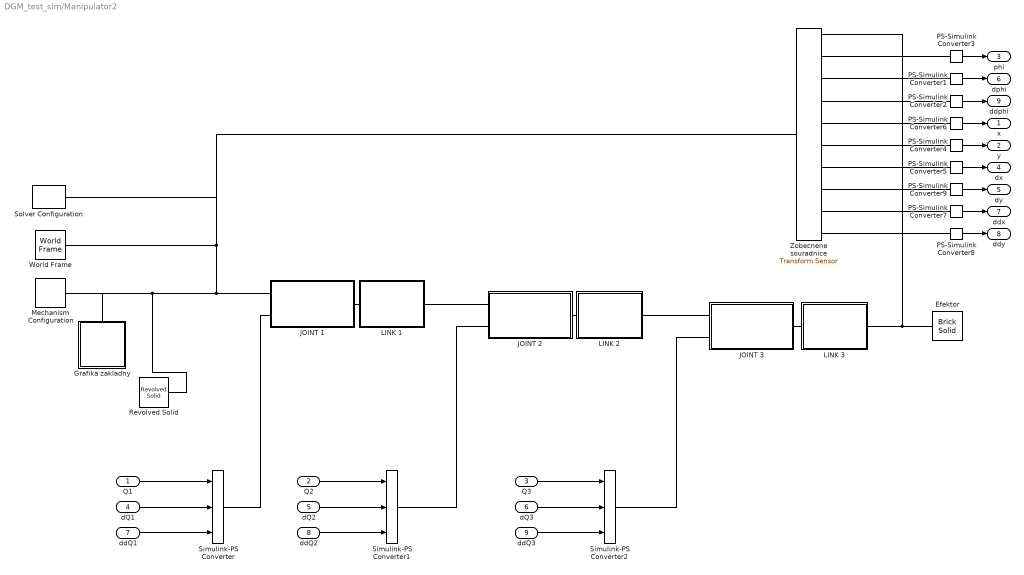
== system DGM_test_sim/Manipulator2 ==
  Q1 : Inport
  Q2 : Inport  Port=2
  Q3 : Inport  Port=3
  dQ1 : Inport  Port=4
  dQ2 : Inport  Port=5
  dQ3 : Inport  Port=6
  ddQ1 : Inport  Port=7
  ddQ2 : Inport  Port=8
  ddQ3 : Inport  Port=9
  Efektor : sm_lib/Body Elements/Brick Solid  GraphicAmbientColor=[0.15 0.15 0.15 1.0]  BasedOnType=Density  BrickDimensions=[0.1 0.1 0.1]  BrickDimensionUnits=m  CenterOfMass=[0 0 0]  CenterOfMassUnits=m  GraphicDiffuseColor=[0.5 0.5 0.5]  Density=1000  DensityUnits=kg/m^3  DoExposeReferenceFrame=on  GraphicEmissiveColor=[0.0 0.0 0.0 1.0]  ExportEntireGeometry=off  SerializedFrames=<Frames/>  MarkerShape=Sphere  MarkerSize=10  GraphicType=FromGeometry  InertiaType=CalculateFromGeometry  Mass=1  MassUnits=kg  MomentsOfInertia=[1 1 1]  MomentsOfInertiaUnits=kg*m^2  GraphicOpacity=1.0  ProductsOfInertia=[0 0 0]  ProductsOfInertiaUnits=kg*m^2  GraphicShininess=75  GraphicSpecularColor=[0.5 0.5 0.5 1.0]  GraphicVisPropType=SimpleVisualProperties
  Grafika zakladny : Subsystem
  JOINT 1 : Subsystem
  JOINT 2 : Subsystem
  JOINT 3 : Subsystem
  LINK 1 : Subsystem
  LINK 2 : Subsystem
  LINK 3 : Subsystem
  Mechanism Configuration : sm_lib/Utilities/Mechanism Configuration  UniformGravity=Constant  GravityVector=[0 0 -9.80665]  GravityUnits=m/s^2  LinearizationDelta=0.001
  PS-Simulink Converter{1..9} (9 alike) : nesl_utility/PS-Simulink Converter  PhysicalDomain=network_engine_domain  SubClassName=ps_output  LeftPortType=input  RightPortType=output  PseudoPeriodic=off  Frequencies=[]  Unit=inherit  AffineConversion=off
      settings: SourceProductBaseCode=PW,SS
  Revolved Solid : sm_lib/Body Elements/Revolved Solid  GraphicAmbientColor=[0.15 0.15 0.15 1.0]  BasedOnType=Density  CenterOfMass=[0 0 0]  CenterOfMassUnits=m  GraphicDiffuseColor=[0.5 0.5 0.5]  ExportConvexHullGeometry=off  Density=1000  DensityUnits=kg/m^3  DoExposeReferenceFrame=on  GraphicEmissiveColor=[0.0 0.0 0.0 1.0]  ExportEntireGeometry=off  SerializedFrames=<Frames/>  MarkerShape=Sphere  MarkerSize=10  GraphicType=FromGeometry  InertiaType=CalculateFromGeometry  Mass=1  MassUnits=kg  MomentsOfInertia=[1 1 1]  MomentsOfInertiaUnits=kg*m^2  GraphicOpacity=0.2  ProductsOfInertia=[0 0 0]  ProductsOfInertiaUnits=kg*m^2  RevolutionCrossSection=[r 0.01; r -0.01; R -0.01; R 0.01]  RevolutionCrossSectionUnits=m  RevolutionAngle=180  RevolutionAngleUnits=deg  RevolutionExtent=Full  GraphicShininess=75  GraphicSpecularColor=[0.5 0.5 0.5 1.0]  GraphicVisPropType=SimpleVisualProperties
  Simulink-PS Converter : nesl_utility/Simulink-PS Converter  PhysicalDomain=network_engine_domain  SubClassName=ps_input  LeftPortType=input  RightPortType=output  PseudoPeriodic=off  Frequencies=[]  NoiseDistribution=none  NoiseParameters=[]  Unit=1  AffineConversion=off  FilteringAndDerivatives=provide  SimscapeFilterOrder=2  InputFilterTimeConstant=0.001  UdotUserProvided=2
      settings: SourceProductBaseCode=PW,SS
  Simulink-PS Converter1 : nesl_utility/Simulink-PS Converter  PhysicalDomain=network_engine_domain  SubClassName=ps_input  LeftPortType=input  RightPortType=output  PseudoPeriodic=off  Frequencies=[]  NoiseDistribution=none  NoiseParameters=[]  Unit=1  AffineConversion=off  FilteringAndDerivatives=provide  SimscapeFilterOrder=2  InputFilterTimeConstant=0.001  UdotUserProvided=2
      settings: SourceProductBaseCode=PW,SS
  Simulink-PS Converter2 : nesl_utility/Simulink-PS Converter  PhysicalDomain=network_engine_domain  SubClassName=ps_input  LeftPortType=input  RightPortType=output  PseudoPeriodic=off  Frequencies=[]  NoiseDistribution=none  NoiseParameters=[]  Unit=1  AffineConversion=off  FilteringAndDerivatives=provide  SimscapeFilterOrder=2  InputFilterTimeConstant=0.001  UdotUserProvided=2
      settings: SourceProductBaseCode=PW,SS
  Solver Configuration : nesl_utility/Solver Configuration  PhysicalDomain=network_engine_domain  SubClassName=solver  LeftPortType=input  RightPortType=generic  Tones=[]  Harmonics=[]  SimulateNoise=off  Profile=off  UseLocalSampling=off  EnableSwitchedLinearOptims=on  FrequencyDomain=off  UseCCode=off  RelTol=0.001  AbsTol=1e-06  MinStep=1e-09  ToWorkspace=off  RevertToSquareIcSolve=off  NumHomotopyIterations=100  PhasorMode=off  PhasorModeNumHarmonics=1  DoDC=off  ResidualTolerance=1e-09  UseLocalSolver=off  LocalSolverChoice=NE_BACKWARD_EULER_ADVANCER  LocalSolverSampleTime=0.001  DoFixedCost=off  MaxNonlinIter=3  MaxModeIter=2  LinearAlgebra=auto  EquationFormulation=NE_TIME_EF  DelaysMemoryBudget=1024  AutomaticFiltering=on  FilteringTimeConstant=0.001  PartitionStorageMethod=AS_NEEDED  PartitionMemoryBudget=1024  PartitionMethod=ROBUST
      settings: SourceProductBaseCode=PW,SS
  World Frame : sm_lib/Frames and Transforms/World Frame
  Zobecnene souradnice : sm_lib/Frames and Transforms/Transform Sensor  MeasurementFrame=World  SenseAngle=on  SenseAxis=off  SenseAngle1=off  SenseAngle2=off  SenseAngle3=off  SenseQ=off  SenseR=off  SenseOmegaX=off  SenseOmegaY=off  SenseOmegaZ=on  SenseOmega1=off  SenseOmega2=off  SenseOmega3=off  SenseQDot=off  SenseRDot=off  SenseAlphaX=off  SenseAlphaY=off  SenseAlphaZ=on  SenseAlpha1=off  SenseAlpha2=off  SenseAlpha3=off  SenseQDDot=off  SenseRDDot=off  SenseX=on  SenseY=on  SenseZ=off  SenseRad=off  SenseAzim=off  SenseDist=off  SenseInc=off  SenseXDot=on  SenseYDot=on  SenseZDot=off  SenseRadDot=off  SenseAzimDot=off  SenseDistDot=off  SenseIncDot=off  SenseXDDot=on  SenseYDDot=on  SenseZDDot=off  SenseRadDDot=off  SenseAzimDDot=off  SenseDistDDot=off  SenseIncDDot=off
  x : Outport
  y : Outport  Port=2
  phi : Outport  Port=3
  dx : Outport  Port=4
  dy : Outport  Port=5
  dphi : Outport  Port=6
  ddx : Outport  Port=7
  ddy : Outport  Port=8
  ddphi : Outport  Port=9
  wires:
  PS-Simulink Converter2/1 -> ddphi/1
  dQ1/1 -> Simulink-PS Converter/2
  Q1/1 -> Simulink-PS Converter/1
  ddQ1/1 -> Simulink-PS Converter/3
  Q2/1 -> Simulink-PS Converter1/1
  ddQ2/1 -> Simulink-PS Converter1/3
  Q3/1 -> Simulink-PS Converter2/1
  dQ3/1 -> Simulink-PS Converter2/2
  ddQ3/1 -> Simulink-PS Converter2/3
  dQ2/1 -> Simulink-PS Converter1/2
  PS-Simulink Converter6/1 -> x/1
  PS-Simulink Converter5/1 -> dx/1
  PS-Simulink Converter7/1 -> ddx/1
  PS-Simulink Converter4/1 -> y/1
  PS-Simulink Converter3/1 -> phi/1
  PS-Simulink Converter1/1 -> dphi/1
  PS-Simulink Converter9/1 -> dy/1
  PS-Simulink Converter8/1 -> ddy/1
  connections:
  Zobecnene souradnice/RConn1 -- Efektor/RConn1 -- LINK 3/RConn1
  Zobecnene souradnice/RConn2 -- PS-Simulink Converter3/LConn1
  Zobecnene souradnice/RConn4 -- PS-Simulink Converter2/LConn1
  PS-Simulink Converter1/LConn1 -- Zobecnene souradnice/RConn3
  Revolved Solid/RConn1 -- Mechanism Configuration/RConn1 -- Grafika zakladny/LConn1 -- JOINT 1/LConn1 -- World Frame/RConn1 -- Solver Configuration/RConn1 -- Zobecnene souradnice/LConn1
  LINK 1/LConn1 -- JOINT 1/RConn1
  JOINT 1/LConn2 -- Simulink-PS Converter/RConn1
  JOINT 2/LConn1 -- LINK 1/RConn1
  JOINT 2/RConn1 -- LINK 2/LConn1
  JOINT 3/LConn1 -- LINK 2/RConn1
  JOINT 3/RConn1 -- LINK 3/LConn1
  Simulink-PS Converter1/RConn1 -- JOINT 2/LConn2
  Simulink-PS Converter2/RConn1 -- JOINT 3/LConn2
  Zobecnene souradnice/RConn6 -- PS-Simulink Converter4/LConn1
  Zobecnene souradnice/RConn5 -- PS-Simulink Converter6/LConn1
  Zobecnene souradnice/RConn7 -- PS-Simulink Converter5/LConn1
  Zobecnene souradnice/RConn9 -- PS-Simulink Converter7/LConn1
  Zobecnene souradnice/RConn8 -- PS-Simulink Converter9/LConn1
  Zobecnene souradnice/RConn10 -- PS-Simulink Converter8/LConn1

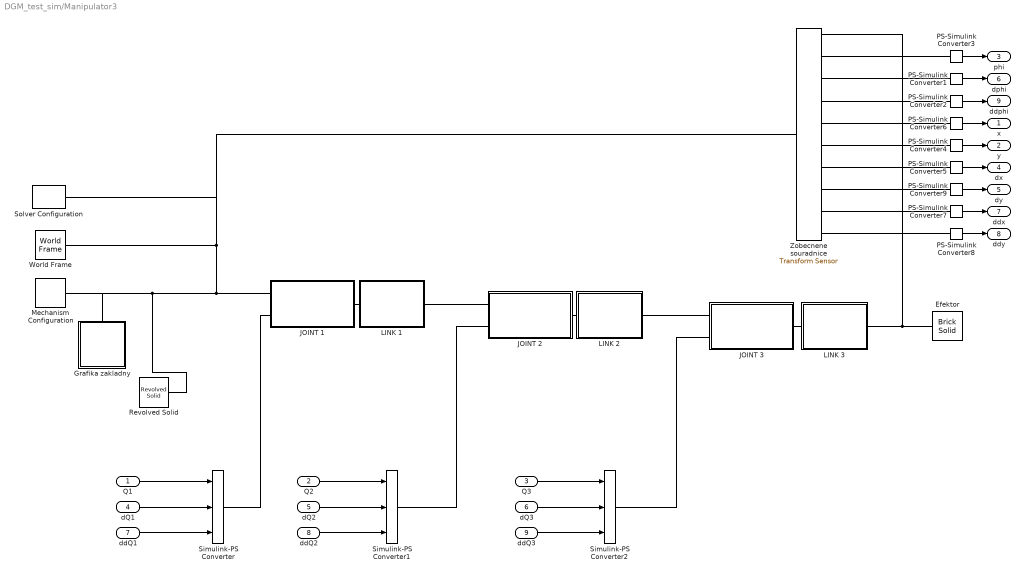
== system DGM_test_sim/Manipulator3 ==
  Q1 : Inport
  Q2 : Inport  Port=2
  Q3 : Inport  Port=3
  dQ1 : Inport  Port=4
  dQ2 : Inport  Port=5
  dQ3 : Inport  Port=6
  ddQ1 : Inport  Port=7
  ddQ2 : Inport  Port=8
  ddQ3 : Inport  Port=9
  Efektor : sm_lib/Body Elements/Brick Solid  GraphicAmbientColor=[0.15 0.15 0.15 1.0]  BasedOnType=Density  BrickDimensions=[0.1 0.1 0.1]  BrickDimensionUnits=m  CenterOfMass=[0 0 0]  CenterOfMassUnits=m  GraphicDiffuseColor=[0.5 0.5 0.5]  Density=1000  DensityUnits=kg/m^3  DoExposeReferenceFrame=on  GraphicEmissiveColor=[0.0 0.0 0.0 1.0]  ExportEntireGeometry=off  SerializedFrames=<Frames/>  MarkerShape=Sphere  MarkerSize=10  GraphicType=FromGeometry  InertiaType=CalculateFromGeometry  Mass=1  MassUnits=kg  MomentsOfInertia=[1 1 1]  MomentsOfInertiaUnits=kg*m^2  GraphicOpacity=1.0  ProductsOfInertia=[0 0 0]  ProductsOfInertiaUnits=kg*m^2  GraphicShininess=75  GraphicSpecularColor=[0.5 0.5 0.5 1.0]  GraphicVisPropType=SimpleVisualProperties
  Grafika zakladny : Subsystem
  JOINT 1 : Subsystem
  JOINT 2 : Subsystem
  JOINT 3 : Subsystem
  LINK 1 : Subsystem
  LINK 2 : Subsystem
  LINK 3 : Subsystem
  Mechanism Configuration : sm_lib/Utilities/Mechanism Configuration  UniformGravity=Constant  GravityVector=[0 0 -9.80665]  GravityUnits=m/s^2  LinearizationDelta=0.001
  PS-Simulink Converter{1..9} (9 alike) : nesl_utility/PS-Simulink Converter  PhysicalDomain=network_engine_domain  SubClassName=ps_output  LeftPortType=input  RightPortType=output  PseudoPeriodic=off  Frequencies=[]  Unit=inherit  AffineConversion=off
      settings: SourceProductBaseCode=PW,SS
  Revolved Solid : sm_lib/Body Elements/Revolved Solid  GraphicAmbientColor=[0.15 0.15 0.15 1.0]  BasedOnType=Density  CenterOfMass=[0 0 0]  CenterOfMassUnits=m  GraphicDiffuseColor=[0.5 0.5 0.5]  ExportConvexHullGeometry=off  Density=1000  DensityUnits=kg/m^3  DoExposeReferenceFrame=on  GraphicEmissiveColor=[0.0 0.0 0.0 1.0]  ExportEntireGeometry=off  SerializedFrames=<Frames/>  MarkerShape=Sphere  MarkerSize=10  GraphicType=FromGeometry  InertiaType=CalculateFromGeometry  Mass=1  MassUnits=kg  MomentsOfInertia=[1 1 1]  MomentsOfInertiaUnits=kg*m^2  GraphicOpacity=0.2  ProductsOfInertia=[0 0 0]  ProductsOfInertiaUnits=kg*m^2  RevolutionCrossSection=[r 0.01; r -0.01; R -0.01; R 0.01]  RevolutionCrossSectionUnits=m  RevolutionAngle=180  RevolutionAngleUnits=deg  RevolutionExtent=Full  GraphicShininess=75  GraphicSpecularColor=[0.5 0.5 0.5 1.0]  GraphicVisPropType=SimpleVisualProperties
  Simulink-PS Converter : nesl_utility/Simulink-PS Converter  PhysicalDomain=network_engine_domain  SubClassName=ps_input  LeftPortType=input  RightPortType=output  PseudoPeriodic=off  Frequencies=[]  NoiseDistribution=none  NoiseParameters=[]  Unit=1  AffineConversion=off  FilteringAndDerivatives=provide  SimscapeFilterOrder=2  InputFilterTimeConstant=0.001  UdotUserProvided=2
      settings: SourceProductBaseCode=PW,SS
  Simulink-PS Converter1 : nesl_utility/Simulink-PS Converter  PhysicalDomain=network_engine_domain  SubClassName=ps_input  LeftPortType=input  RightPortType=output  PseudoPeriodic=off  Frequencies=[]  NoiseDistribution=none  NoiseParameters=[]  Unit=1  AffineConversion=off  FilteringAndDerivatives=provide  SimscapeFilterOrder=2  InputFilterTimeConstant=0.001  UdotUserProvided=2
      settings: SourceProductBaseCode=PW,SS
  Simulink-PS Converter2 : nesl_utility/Simulink-PS Converter  PhysicalDomain=network_engine_domain  SubClassName=ps_input  LeftPortType=input  RightPortType=output  PseudoPeriodic=off  Frequencies=[]  NoiseDistribution=none  NoiseParameters=[]  Unit=1  AffineConversion=off  FilteringAndDerivatives=provide  SimscapeFilterOrder=2  InputFilterTimeConstant=0.001  UdotUserProvided=2
      settings: SourceProductBaseCode=PW,SS
  Solver Configuration : nesl_utility/Solver Configuration  PhysicalDomain=network_engine_domain  SubClassName=solver  LeftPortType=input  RightPortType=generic  Tones=[]  Harmonics=[]  SimulateNoise=off  Profile=off  UseLocalSampling=off  EnableSwitchedLinearOptims=on  FrequencyDomain=off  UseCCode=off  RelTol=0.001  AbsTol=1e-06  MinStep=1e-09  ToWorkspace=off  RevertToSquareIcSolve=off  NumHomotopyIterations=100  PhasorMode=off  PhasorModeNumHarmonics=1  DoDC=off  ResidualTolerance=1e-09  UseLocalSolver=off  LocalSolverChoice=NE_BACKWARD_EULER_ADVANCER  LocalSolverSampleTime=0.001  DoFixedCost=off  MaxNonlinIter=3  MaxModeIter=2  LinearAlgebra=auto  EquationFormulation=NE_TIME_EF  DelaysMemoryBudget=1024  AutomaticFiltering=on  FilteringTimeConstant=0.001  PartitionStorageMethod=AS_NEEDED  PartitionMemoryBudget=1024  PartitionMethod=ROBUST
      settings: SourceProductBaseCode=PW,SS
  World Frame : sm_lib/Frames and Transforms/World Frame
  Zobecnene souradnice : sm_lib/Frames and Transforms/Transform Sensor  MeasurementFrame=World  SenseAngle=on  SenseAxis=off  SenseAngle1=off  SenseAngle2=off  SenseAngle3=off  SenseQ=off  SenseR=off  SenseOmegaX=off  SenseOmegaY=off  SenseOmegaZ=on  SenseOmega1=off  SenseOmega2=off  SenseOmega3=off  SenseQDot=off  SenseRDot=off  SenseAlphaX=off  SenseAlphaY=off  SenseAlphaZ=on  SenseAlpha1=off  SenseAlpha2=off  SenseAlpha3=off  SenseQDDot=off  SenseRDDot=off  SenseX=on  SenseY=on  SenseZ=off  SenseRad=off  SenseAzim=off  SenseDist=off  SenseInc=off  SenseXDot=on  SenseYDot=on  SenseZDot=off  SenseRadDot=off  SenseAzimDot=off  SenseDistDot=off  SenseIncDot=off  SenseXDDot=on  SenseYDDot=on  SenseZDDot=off  SenseRadDDot=off  SenseAzimDDot=off  SenseDistDDot=off  SenseIncDDot=off
  x : Outport
  y : Outport  Port=2
  phi : Outport  Port=3
  dx : Outport  Port=4
  dy : Outport  Port=5
  dphi : Outport  Port=6
  ddx : Outport  Port=7
  ddy : Outport  Port=8
  ddphi : Outport  Port=9
  wires:
  PS-Simulink Converter2/1 -> ddphi/1
  dQ1/1 -> Simulink-PS Converter/2
  Q1/1 -> Simulink-PS Converter/1
  ddQ1/1 -> Simulink-PS Converter/3
  Q2/1 -> Simulink-PS Converter1/1
  ddQ2/1 -> Simulink-PS Converter1/3
  Q3/1 -> Simulink-PS Converter2/1
  dQ3/1 -> Simulink-PS Converter2/2
  ddQ3/1 -> Simulink-PS Converter2/3
  dQ2/1 -> Simulink-PS Converter1/2
  PS-Simulink Converter6/1 -> x/1
  PS-Simulink Converter5/1 -> dx/1
  PS-Simulink Converter7/1 -> ddx/1
  PS-Simulink Converter4/1 -> y/1
  PS-Simulink Converter3/1 -> phi/1
  PS-Simulink Converter1/1 -> dphi/1
  PS-Simulink Converter9/1 -> dy/1
  PS-Simulink Converter8/1 -> ddy/1
  connections:
  Zobecnene souradnice/RConn1 -- Efektor/RConn1 -- LINK 3/RConn1
  Zobecnene souradnice/RConn2 -- PS-Simulink Converter3/LConn1
  Zobecnene souradnice/RConn4 -- PS-Simulink Converter2/LConn1
  PS-Simulink Converter1/LConn1 -- Zobecnene souradnice/RConn3
  Revolved Solid/RConn1 -- Mechanism Configuration/RConn1 -- Grafika zakladny/LConn1 -- JOINT 1/LConn1 -- World Frame/RConn1 -- Solver Configuration/RConn1 -- Zobecnene souradnice/LConn1
  LINK 1/LConn1 -- JOINT 1/RConn1
  JOINT 1/LConn2 -- Simulink-PS Converter/RConn1
  JOINT 2/LConn1 -- LINK 1/RConn1
  JOINT 2/RConn1 -- LINK 2/LConn1
  JOINT 3/LConn1 -- LINK 2/RConn1
  JOINT 3/RConn1 -- LINK 3/LConn1
  Simulink-PS Converter1/RConn1 -- JOINT 2/LConn2
  Simulink-PS Converter2/RConn1 -- JOINT 3/LConn2
  Zobecnene souradnice/RConn6 -- PS-Simulink Converter4/LConn1
  Zobecnene souradnice/RConn5 -- PS-Simulink Converter6/LConn1
  Zobecnene souradnice/RConn7 -- PS-Simulink Converter5/LConn1
  Zobecnene souradnice/RConn9 -- PS-Simulink Converter7/LConn1
  Zobecnene souradnice/RConn8 -- PS-Simulink Converter9/LConn1
  Zobecnene souradnice/RConn10 -- PS-Simulink Converter8/LConn1
